simulink model "Testbench_Algorithm"  (R2019b)
settings: Solver=VariableStepAuto  StartTime=0.0  StopTime=10.0  RelTol=1e-3
values from neighbouring files (symbols this model uses):
  bo = b0/(c*a1)    [otpADRC.m]
  wc = 1/(c*a1)    [otpADRC.m]
undefined symbols (not defined in the file or in its folder): A, B, C, D, obs
libraries: simulink x1
settings Model: Creator=didi  LastModifiedBy=didi

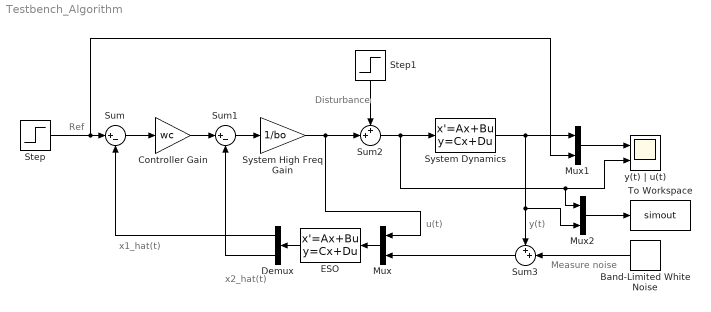
== system Testbench_Algorithm ==
  note: y(t)
  note: x2_hat(t)
  note: Measure noise
  note: Ref
  note: u(t)
  note: Disturbance
  note: x1_hat(t)
  Band-Limited White Noise : simulink/Sources/Band-Limited White Noise  Cov=[0.000001]  Ts=0.76  seed=[23341]
  Controller Gain : Gain  Gain=wc
  Demux : Demux  Outputs=2
  ESO : StateSpace  A=obs.A  B=obs.B  C=obs.C  D=obs.D  InitialCondition=0
  Mux : Mux  Inputs=2
  Mux1 : Mux  Inputs=2
  Mux2 : Mux  Inputs=2
  Step : Step  SampleTime=0
  Step1 : Step  Time=5  After=5  SampleTime=0
  Sum : Sum  Inputs=|+-
  Sum1 : Sum  Inputs=|+-
  Sum2 : Sum  Inputs=++|
  Sum3 : Sum  Inputs=++|
  System Dynamics : StateSpace  A=A  B=B  C=C  D=D  InitialCondition=0
  System High Freq Gain : Gain  Gain=1/bo
  To Workspace : ToWorkspace  VariableName=simout  SaveFormat=Timeseries  SampleTime=-1
  y(t) | u(t) : Scope  NumInputPorts=2
  wires:
  Controller Gain/1 -> Sum1/1
  System Dynamics/1 -> Mux2/2, Sum3/1, Mux1/1
  Step/1 -> Mux1/2, Sum/1
  Sum/1 -> Controller Gain/1
  Sum3/1 -> Mux/2
  Mux/1 -> ESO/1
  ESO/1 -> Demux/1
  Demux/2 -> Sum1/2
  Sum2/1 -> Mux2/1, y(t) | u(t)/2, System Dynamics/1
  Demux/1 -> Sum/2
  Mux1/1 -> y(t) | u(t)/1
  System High Freq Gain/1 -> Mux/1, Sum2/2
  Sum1/1 -> System High Freq Gain/1
  Step1/1 -> Sum2/1
  Band-Limited White Noise/1 -> Sum3/2
  Mux2/1 -> To Workspace/1
